simulink model "Parachute_StateSpace"  (R2018a)
settings: Solver=VariableStepAuto  StartTime=0.0  StopTime=4  RelTol=1e-3
values from neighbouring files (symbols this model uses):
  A = [-Bp/Mp 0 -Kr/Mp Kr/Mp ... (first row only)    [Main.m]
  B = [Mp;Mj;0;0]    [Main.m]
  C = [1 1 0 0]    [Main.m]
  D = 0    [Main.m]
  X0 = [20; 20; 0; 0]    [Main.m]
settings Model: Creator=Eduardo  LastModifiedBy=Eduardo Montilva

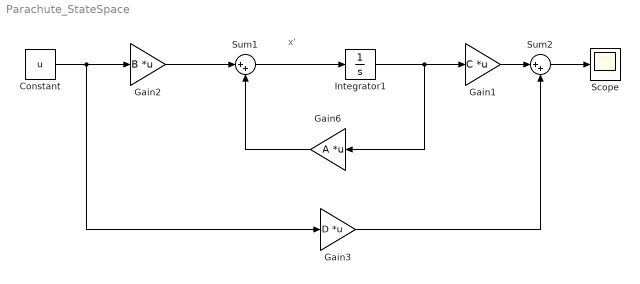
== system Parachute_StateSpace ==
  note: x'
  Constant : Constant  Value=u
  Gain1 : Gain  Gain=C  Multiplication=Matrix(K*u)
  Gain2 : Gain  Gain=B  Multiplication=Matrix(K*u)
  Gain3 : Gain  Gain=D  Multiplication=Matrix(K*u)
  Gain6 : Gain  Gain=A  Multiplication=Matrix(K*u)
  Integrator1 : Integrator  InitialCondition=X0
  Scope : Scope
  Sum1 : Sum  Inputs=|++
  Sum2 : Sum  Inputs=|++
  wires:
  Gain6/1 -> Sum1/2
  Constant/1 -> Gain3/1, Gain2/1
  Gain2/1 -> Sum1/1
  Sum1/1 -> Integrator1/1
  Integrator1/1 -> Gain1/1, Gain6/1
  Gain1/1 -> Sum2/1
  Gain3/1 -> Sum2/2
  Sum2/1 -> Scope/1
